simulink model "Model_3RC"  (R2022b)
settings: Solver=FixedStepAuto  StartTime=0.0  StopTime=10000  FixedStep=1  RelTol=1e-3
undefined symbols (not defined in the file): OCV, R0, R1, R2, R3, SOC_levels, tau1, tau2, tau3
settings Model: Creator=frederikvanmaele  LastModifiedBy=AdministratorDevice
settings DebuggingCC: UnconnectedInputMsg=warning  UnconnectedOutputMsg=warning  UnconnectedLineMsg=warning
settings ModelReferenceCC: EnableRefExpFcnMdlSchedulingChecks=on
settings RTWCC: DLArmComputeVersion=19.05

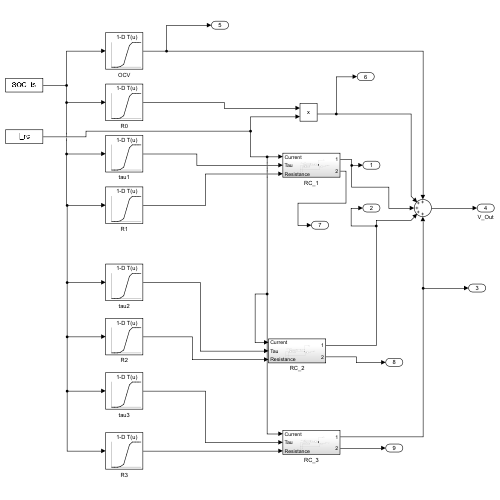
[thumbnail: Simulink's stored preview of the top-level diagram]
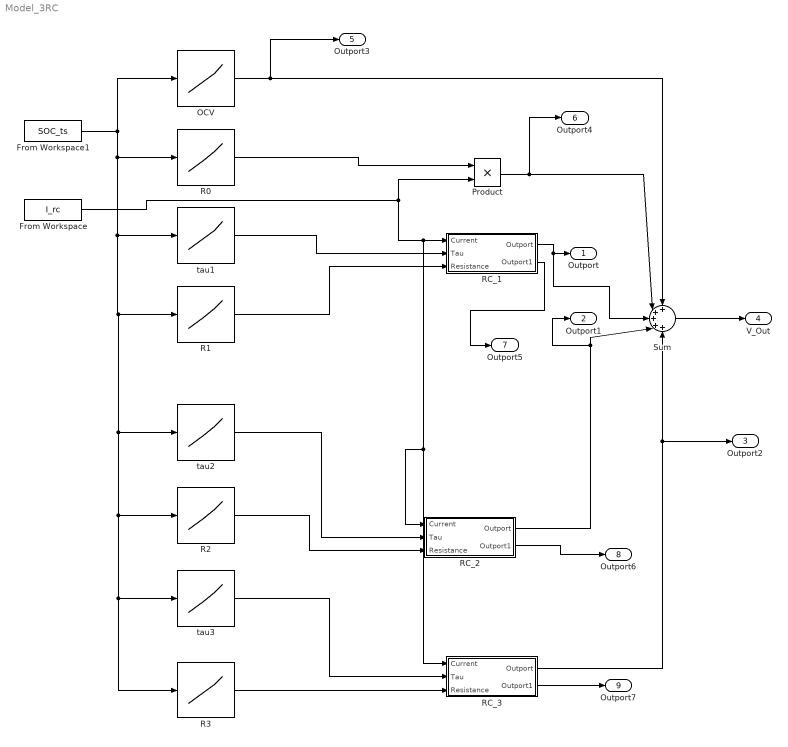
== system Model_3RC ==
  From Workspace : FromWorkspace  VariableName=I_rc
  From Workspace1 : FromWorkspace  VariableName=SOC_ts
  OCV : Lookup_n-D  NumberOfTableDimensions=1  BreakpointsForDimension1=SOC_levels  BeginIndexSearchUsingPreviousIndexResult=on  Table=OCV  UseLastTableValue=on  InternalRulePriority=Speed  OutDataTypeStr=Inherit: Inherit via back propagation  RndMeth=Simplest
  Product : Product
  R0 : Lookup_n-D  NumberOfTableDimensions=1  BreakpointsForDimension1=SOC_levels  BeginIndexSearchUsingPreviousIndexResult=on  Table=R0  ExtrapMethod=Clip  UseLastTableValue=on  InternalRulePriority=Speed  RndMeth=Simplest
  R1 : Lookup_n-D  NumberOfTableDimensions=1  BreakpointsForDimension1=SOC_levels  BeginIndexSearchUsingPreviousIndexResult=on  Table=R1  ExtrapMethod=Clip  UseLastTableValue=on  InternalRulePriority=Speed  RndMeth=Simplest
  R2 : Lookup_n-D  NumberOfTableDimensions=1  BreakpointsForDimension1=SOC_levels  BeginIndexSearchUsingPreviousIndexResult=on  Table=R2  ExtrapMethod=Clip  UseLastTableValue=on  InternalRulePriority=Speed  RndMeth=Simplest
  R3 : Lookup_n-D  NumberOfTableDimensions=1  BreakpointsForDimension1=SOC_levels  BeginIndexSearchUsingPreviousIndexResult=on  Table=R3  ExtrapMethod=Clip  UseLastTableValue=on  InternalRulePriority=Speed  RndMeth=Simplest
  RC_1 : Subsystem
  RC_2 : Subsystem
  RC_3 : Subsystem
  Sum : Sum  Inputs=+++++
  tau1 : Lookup_n-D  NumberOfTableDimensions=1  BreakpointsForDimension1=SOC_levels  BeginIndexSearchUsingPreviousIndexResult=on  Table=tau1  ExtrapMethod=Clip  UseLastTableValue=on  InternalRulePriority=Speed  RndMeth=Simplest
  tau2 : Lookup_n-D  NumberOfTableDimensions=1  BreakpointsForDimension1=SOC_levels  BeginIndexSearchUsingPreviousIndexResult=on  Table=tau2  ExtrapMethod=Clip  UseLastTableValue=on  InternalRulePriority=Speed  RndMeth=Simplest
  tau3 : Lookup_n-D  NumberOfTableDimensions=1  BreakpointsForDimension1=SOC_levels  BeginIndexSearchUsingPreviousIndexResult=on  Table=tau3  ExtrapMethod=Clip  UseLastTableValue=on  InternalRulePriority=Speed  RndMeth=Simplest
  Outport : Outport
  Outport1 : Outport  Port=2
  Outport2 : Outport  Port=3
  V_Out : Outport  Port=4
  Outport3 : Outport  Port=5
  Outport4 : Outport  Port=6
  Outport5 : Outport  Port=7
  Outport6 : Outport  Port=8
  Outport7 : Outport  Port=9
  wires:
  R1/1 -> RC_1/3(Resistance)
  tau1/1 -> RC_1/2(Tau)
  From Workspace/1 -> RC_1/1(Current), RC_3/1(Current), RC_2/1(Current), Product/2
  RC_1/1(Outport) -> Sum/3, Outport/1
  R2/1 -> RC_2/3(Resistance)
  OCV/1 -> Outport3/1, Sum/1
  Sum/1 -> V_Out/1
  From Workspace1/1 -> R0/1, tau1/1, R1/1, tau2/1, R2/1, R3/1, tau3/1, OCV/1
  R0/1 -> Product/1
  Product/1 -> Outport4/1, Sum/2
  tau2/1 -> RC_2/2(Tau)
  tau3/1 -> RC_3/2(Tau)
  R3/1 -> RC_3/3(Resistance)
  RC_1/2(Outport1) -> Outport5/1
  RC_3/2(Outport1) -> Outport7/1
  RC_3/1(Outport) -> Outport2/1, Sum/5
  RC_2/2(Outport1) -> Outport6/1
  RC_2/1(Outport) -> Outport1/1, Sum/4

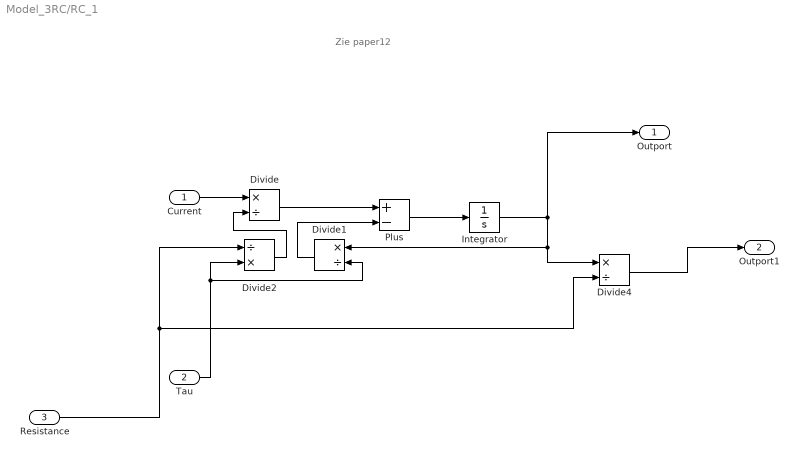
== system Model_3RC/RC_1 ==
  note: Zie paper12
  Current : Inport
  Tau : Inport  Port=2
  Resistance : Inport  Port=3
  Divide : Product  Inputs=*/
  Divide1 : Product  Inputs=*/
  Divide2 : Product  Inputs=/*
  Divide4 : Product  Inputs=*/
  Integrator : Integrator
  Plus : Sum  Inputs=+-
  Outport : Outport
  Outport1 : Outport  Port=2
  wires:
  Tau/1 -> Divide2/2, Divide1/2
  Divide/1 -> Plus/1
  Plus/1 -> Integrator/1
  Current/1 -> Divide/1
  Divide1/1 -> Plus/2
  Resistance/1 -> Divide4/2, Divide2/1
  Divide2/1 -> Divide/2
  Integrator/1 -> Divide4/1, Divide1/1, Outport/1
  Divide4/1 -> Outport1/1

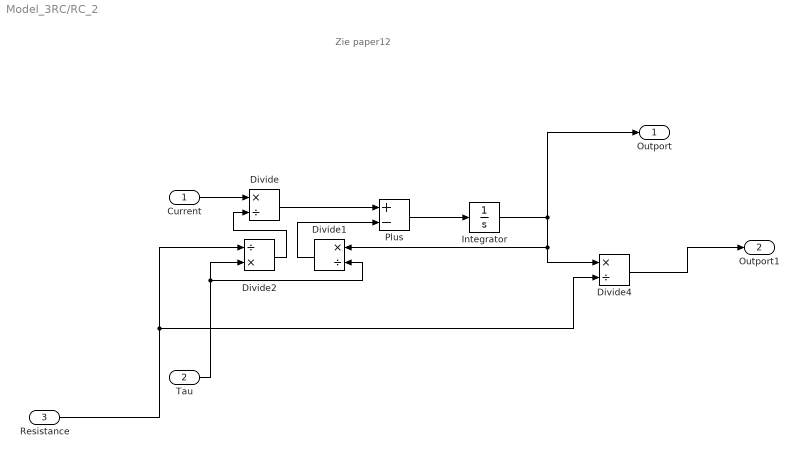
== system Model_3RC/RC_2 ==
  note: Zie paper12
  Current : Inport
  Tau : Inport  Port=2
  Resistance : Inport  Port=3
  Divide : Product  Inputs=*/
  Divide1 : Product  Inputs=*/
  Divide2 : Product  Inputs=/*
  Divide4 : Product  Inputs=*/
  Integrator : Integrator
  Plus : Sum  Inputs=+-
  Outport : Outport
  Outport1 : Outport  Port=2
  wires:
  Tau/1 -> Divide2/2, Divide1/2
  Divide/1 -> Plus/1
  Plus/1 -> Integrator/1
  Current/1 -> Divide/1
  Divide1/1 -> Plus/2
  Resistance/1 -> Divide4/2, Divide2/1
  Divide2/1 -> Divide/2
  Integrator/1 -> Divide4/1, Divide1/1, Outport/1
  Divide4/1 -> Outport1/1

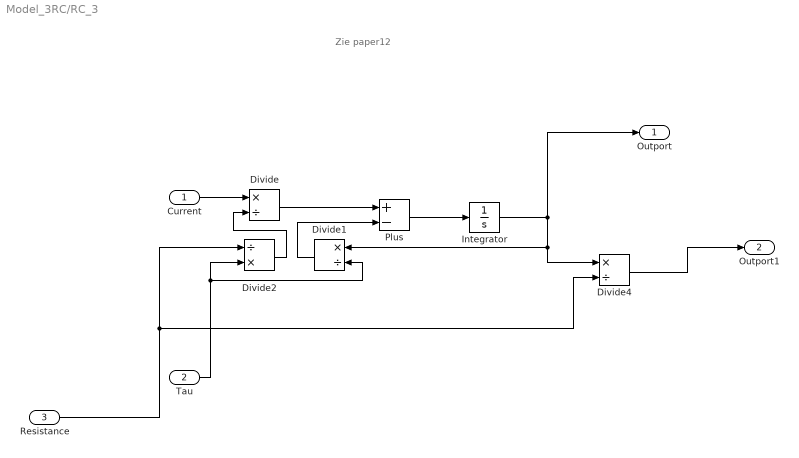
== system Model_3RC/RC_3 ==
  note: Zie paper12
  Current : Inport
  Tau : Inport  Port=2
  Resistance : Inport  Port=3
  Divide : Product  Inputs=*/
  Divide1 : Product  Inputs=*/
  Divide2 : Product  Inputs=/*
  Divide4 : Product  Inputs=*/
  Integrator : Integrator
  Plus : Sum  Inputs=+-
  Outport : Outport
  Outport1 : Outport  Port=2
  wires:
  Tau/1 -> Divide2/2, Divide1/2
  Divide/1 -> Plus/1
  Plus/1 -> Integrator/1
  Current/1 -> Divide/1
  Divide1/1 -> Plus/2
  Resistance/1 -> Divide4/2, Divide2/1
  Divide2/1 -> Divide/2
  Integrator/1 -> Divide4/1, Divide1/1, Outport/1
  Divide4/1 -> Outport1/1
